simulink model "G_complete"  (R2020b)
settings: Solver=VariableStepAuto  StartTime=0.0  StopTime=2  RelTol=1e-9
undefined symbols (not defined in the file): r_step, T_i
libraries: cstblocks x4
settings Model: Creator=jasper  LastModifiedBy=jasper

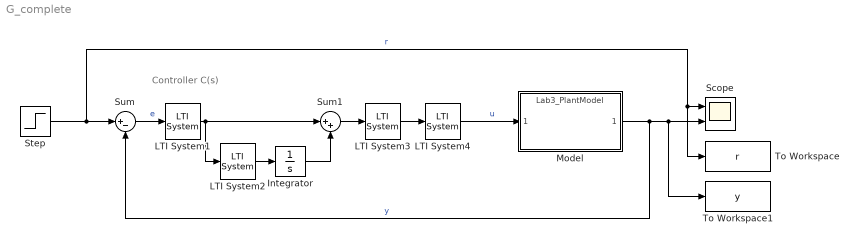
== system G_complete ==
  note: Controller C(s)
  Integrator : Integrator  LimitOutput=on  UpperSaturationLimit=10  LowerSaturationLimit=-10
  LTI System1 : cstblocks/LTI System  sys=K_p  IC=[]
  LTI System2 : cstblocks/LTI System  sys=1/T_i  IC=[]
  LTI System3 : cstblocks/LTI System  sys=G_lead  IC=[]
  LTI System4 : cstblocks/LTI System  sys=G_lpf  IC=[]
  Model : ModelReference  ModelNameDialog=Lab3_PlantModel  SimulationMode=Normal  ModelReferenceVersion=2.1
  Scope : Scope  NumInputPorts=2
  Step : Step  Time=0.1  After=r_step  SampleTime=0
  Sum : Sum  Inputs=|+-
  Sum1 : Sum  Inputs=|++
  To Workspace : ToWorkspace  VariableName=r  SaveFormat=Timeseries  SampleTime=-1
  To Workspace1 : ToWorkspace  VariableName=y  SaveFormat=Timeseries  SampleTime=-1
  wires:
  Step/1 -> Sum/1, Scope/1, To Workspace/1  "r"
  Sum/1 -> LTI System1/1  "e"
  LTI System1/1 -> Sum1/1, LTI System2/1
  LTI System2/1 -> Integrator/1
  Integrator/1 -> Sum1/2
  Sum1/1 -> LTI System3/1
  LTI System3/1 -> LTI System4/1
  LTI System4/1 -> Model/1  "u"
  Model/1 -> To Workspace1/1, Scope/2, Sum/2  "y"
